simulink model "VVI"  (R2020a)
settings: Solver=FixedStepAuto  StartTime=0.0  StopTime=10.0  FixedStep=1e-3  RelTol=1e-3  EnableMultiTasking=on
undefined symbols (not defined in the file): D0, D1, D10, D11, D12, D13, D2, D3, D4, D5, D6, D7, D8, D9, PTA0, PTA1, PTA2, PTB23, PTB9, PTC16, PTC17, PTC2, PTC3, PTC4, PTD0, PTD1, PTD2, PTD3
libraries: frdmk64flib x15
settings Model: ExtModeTrigDuration=5  Creator=abdullah  LastModifiedBy=abdullah
settings OptimizationCC: EnhancedBackFolding=on  PassReuseOutputArgsAs=Individual arguments  ZeroExternalMemoryAtStartup=off  ZeroInternalMemoryAtStartup=off  MaxStackSize=64  OptimizeBlockOrder=speed  DifferentSizesBufferReuse=on  OptimizationCustomize=off  EfficientTunableParamExpr=on
settings DebuggingCC: ParameterTunabilityLossMsg=error
settings HardwareCC: ProdBitPerPointer=32  ProdBitPerSizeT=32  ProdBitPerPtrDiffT=32  ProdLargestAtomicInteger=Long  ProdLargestAtomicFloat=Double  ProdWordSize=32  ProdHWDeviceType=ARM Compatible->ARM Cortex
settings SFSimCC: MATLABDynamicMemAlloc=off
settings RTWCC: SystemTargetFile=ert.tlc  HardwareBoard=NXP FRDM-K64F  TemplateMakefile=ert_default_tmf  Toolchain=GNU Tools for ARM Embedded Processors
settings CodeAppCC: ForceParamTrailComments=on  IgnoreCustomStorageClasses=off  OperatorAnnotations=on  SimulinkDataObjDesc=on  SFDataObjDesc=on  InsertBlockDesc=on

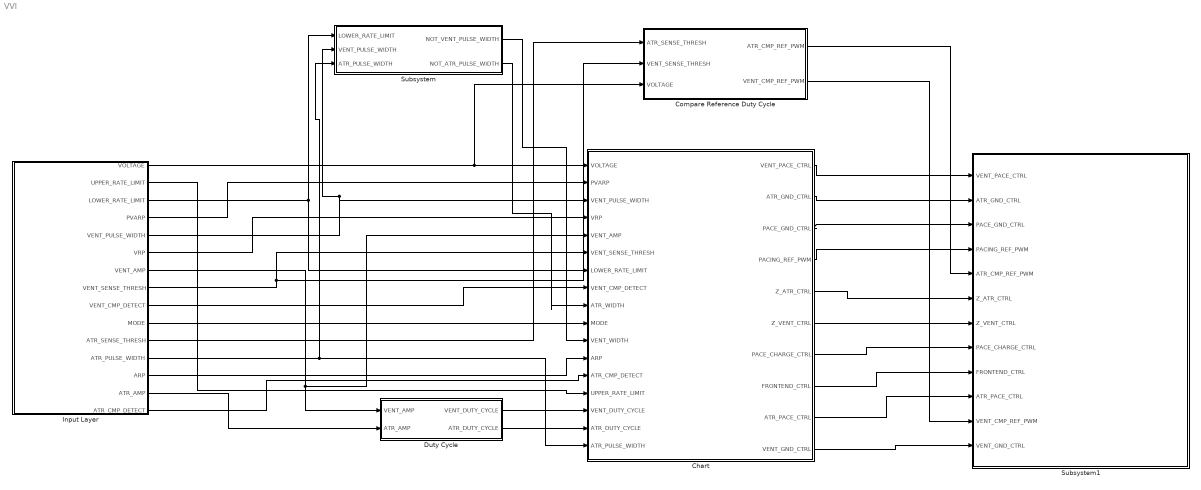
== system VVI ==
  Chart : Stateflow chart  TreatAsAtomicUnit=on
  Compare Reference Duty Cycle : Subsystem
  Duty Cycle : Subsystem
  Input Layer : Subsystem
  Subsystem : Subsystem
  Subsystem1 : Subsystem
  wires:
  Input Layer/1(VOLTAGE) -> Chart/1(VOLTAGE), Compare Reference Duty Cycle/3(VOLTAGE)
  Input Layer/2(UPPER_RATE_LIMIT) -> Chart/14(UPPER_RATE_LIMIT)
  Input Layer/3(LOWER_RATE_LIMIT) -> Subsystem/1(LOWER_RATE_LIMIT), Chart/7(LOWER_RATE_LIMIT)
  Input Layer/4(PVARP) -> Chart/2(PVARP)
  Input Layer/5(VENT_PULSE_WIDTH) -> Subsystem/2(VENT_PULSE_WIDTH), Chart/3(VENT_PULSE_WIDTH)
  Input Layer/6(VRP) -> Chart/4(VRP)
  Input Layer/7(VENT_AMP) -> Duty Cycle/1(VENT_AMP), Chart/5(VENT_AMP)
  Input Layer/8(VENT_SENSE_THRESH) -> Chart/6(VENT_SENSE_THRESH), Compare Reference Duty Cycle/2(VENT_SENSE_THRESH)
  Input Layer/9(VENT_CMP_DETECT) -> Chart/8(VENT_CMP_DETECT)
  Subsystem/1(NOT_VENT_PULSE_WIDTH) -> Chart/11(VENT_WIDTH)
  Chart/1(VENT_PACE_CTRL) -> Subsystem1/1(VENT_PACE_CTRL)
  Chart/2(ATR_GND_CTRL) -> Subsystem1/2(ATR_GND_CTRL)
  Chart/3(PACE_GND_CTRL) -> Subsystem1/3(PACE_GND_CTRL)
  Chart/4(PACING_REF_PWM) -> Subsystem1/4(PACING_REF_PWM)
  Chart/5(Z_ATR_CTRL) -> Subsystem1/6(Z_ATR_CTRL)
  Chart/6(Z_VENT_CTRL) -> Subsystem1/7(Z_VENT_CTRL)
  Chart/7(PACE_CHARGE_CTRL) -> Subsystem1/8(PACE_CHARGE_CTRL)
  Chart/8(FRONTEND_CTRL) -> Subsystem1/9(FRONTEND_CTRL)
  Chart/9(ATR_PACE_CTRL) -> Subsystem1/10(ATR_PACE_CTRL)
  Chart/10(VENT_GND_CTRL) -> Subsystem1/12(VENT_GND_CTRL)
  Duty Cycle/1(VENT_DUTY_CYCLE) -> Chart/15(VENT_DUTY_CYCLE)
  Compare Reference Duty Cycle/1(ATR_CMP_REF_PWM) -> Subsystem1/5(ATR_CMP_REF_PWM)
  Compare Reference Duty Cycle/2(VENT_CMP_REF_PWM) -> Subsystem1/11(VENT_CMP_REF_PWM)
  Input Layer/11(ATR_SENSE_THRESH) -> Compare Reference Duty Cycle/1(ATR_SENSE_THRESH)
  Input Layer/10(MODE) -> Chart/10(MODE)
  Input Layer/12(ATR_PULSE_WIDTH) -> Subsystem/3(ATR_PULSE_WIDTH), Chart/17(ATR_PULSE_WIDTH)
  Subsystem/2(NOT_ATR_PULSE_WIDTH) -> Chart/9(ATR_WIDTH)
  Input Layer/13(ARP) -> Chart/12(ARP)
  Input Layer/14(ATR_AMP) -> Duty Cycle/2(ATR_AMP)
  Duty Cycle/2(ATR_DUTY_CYCLE) -> Chart/16(ATR_DUTY_CYCLE)
  Input Layer/15(ATR_CMP_DETECT) -> Chart/13(ATR_CMP_DETECT)

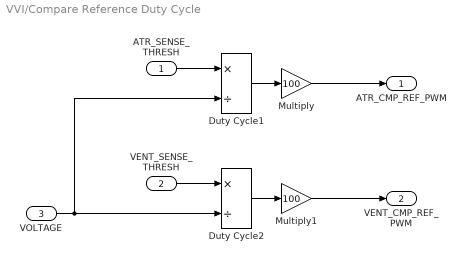
== system VVI/Compare Reference Duty Cycle ==
  ATR_SENSE_THRESH : Inport
  VENT_SENSE_THRESH : Inport  Port=2
  VOLTAGE : Inport  Port=3
  Duty Cycle1 : Product  Inputs=*/
  Duty Cycle2 : Product  Inputs=*/
  Multiply : Gain  Gain=100
  Multiply1 : Gain  Gain=100
  ATR_CMP_REF_PWM : Outport  VectorParamsAs1DForOutWhenUnconnected=off
  VENT_CMP_REF_PWM : Outport  Port=2  VectorParamsAs1DForOutWhenUnconnected=off
  wires:
  Multiply1/1 -> VENT_CMP_REF_PWM/1
  VENT_SENSE_THRESH/1 -> Duty Cycle2/1
  Duty Cycle2/1 -> Multiply1/1
  ATR_SENSE_THRESH/1 -> Duty Cycle1/1
  Duty Cycle1/1 -> Multiply/1
  Multiply/1 -> ATR_CMP_REF_PWM/1
  VOLTAGE/1 -> Duty Cycle1/2, Duty Cycle2/2

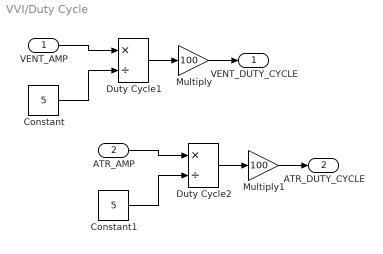
== system VVI/Duty Cycle ==
  VENT_AMP : Inport
  ATR_AMP : Inport  Port=2
  Constant : Constant  Value=5  OutDataTypeStr=single
  Constant1 : Constant  Value=5  OutDataTypeStr=single
  Duty Cycle1 : Product  Inputs=*/
  Duty Cycle2 : Product  Inputs=*/
  Multiply : Gain  Gain=100
  Multiply1 : Gain  Gain=100
  VENT_DUTY_CYCLE : Outport  VectorParamsAs1DForOutWhenUnconnected=off
  ATR_DUTY_CYCLE : Outport  Port=2  VectorParamsAs1DForOutWhenUnconnected=off
  wires:
  Constant/1 -> Duty Cycle1/2
  VENT_AMP/1 -> Duty Cycle1/1
  Duty Cycle1/1 -> Multiply/1
  Multiply/1 -> VENT_DUTY_CYCLE/1
  ATR_AMP/1 -> Duty Cycle2/1
  Multiply1/1 -> ATR_DUTY_CYCLE/1
  Constant1/1 -> Duty Cycle2/2
  Duty Cycle2/1 -> Multiply1/1

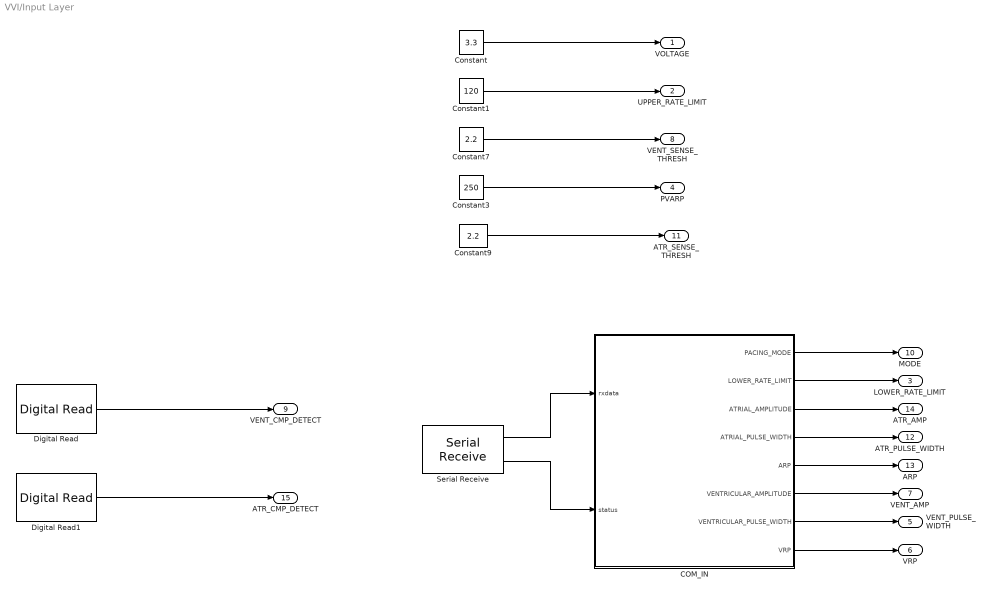
== system VVI/Input Layer ==
  COM_IN : Stateflow chart  TreatAsAtomicUnit=on
  Constant : Constant  Value=3.3  OutDataTypeStr=single
  Constant1 : Constant  Value=120  OutDataTypeStr=uint8
  Constant3 : Constant  Value=250  OutDataTypeStr=uint16
  Constant7 : Constant  Value=2.2  OutDataTypeStr=single
  Constant9 : Constant  Value=2.2  OutDataTypeStr=single
  Digital Read : frdmk64flib/Digital Read  Whichpin=PTC17 (D1)  SampleTime=-1
  Digital Read1 : frdmk64flib/Digital Read  Whichpin=PTC16 (D0)  SampleTime=-1
  Serial Receive : frdmk64flib/Serial Receive  SCIModule=0  Baudrate=uint32(9600)  Parity=None  StopBits=1  HardwareFlowControl=None  ByteOrder=LittleEndian  DataType=uint8  DataLength=24  BlockingMode=off  OutputStatus=on  SampleTime=-1
  VOLTAGE : Outport
  UPPER_RATE_LIMIT : Outport  Port=2
  LOWER_RATE_LIMIT : Outport  Port=3
  PVARP : Outport  Port=4
  VENT_PULSE_WIDTH : Outport  Port=5
  VRP : Outport  Port=6
  VENT_AMP : Outport  Port=7
  VENT_SENSE_THRESH : Outport  Port=8
  VENT_CMP_DETECT : Outport  Port=9
  MODE : Outport  Port=10
  ATR_SENSE_THRESH : Outport  Port=11
  ATR_PULSE_WIDTH : Outport  Port=12
  ARP : Outport  Port=13
  ATR_AMP : Outport  Port=14
  ATR_CMP_DETECT : Outport  Port=15
  wires:
  Serial Receive/1 -> COM_IN/1(rxdata)
  Constant1/1 -> UPPER_RATE_LIMIT/1
  Constant3/1 -> PVARP/1
  Constant/1 -> VOLTAGE/1
  Constant9/1 -> ATR_SENSE_THRESH/1
  Digital Read1/1 -> ATR_CMP_DETECT/1
  Constant7/1 -> VENT_SENSE_THRESH/1
  COM_IN/5(ARP) -> ARP/1
  Digital Read/1 -> VENT_CMP_DETECT/1
  COM_IN/3(ATRIAL_AMPLITUDE) -> ATR_AMP/1
  COM_IN/6(VENTRICULAR_AMPLITUDE) -> VENT_AMP/1
  COM_IN/7(VENTRICULAR_PULSE_WIDTH) -> VENT_PULSE_WIDTH/1
  COM_IN/8(VRP) -> VRP/1
  COM_IN/2(LOWER_RATE_LIMIT) -> LOWER_RATE_LIMIT/1
  COM_IN/4(ATRIAL_PULSE_WIDTH) -> ATR_PULSE_WIDTH/1
  COM_IN/1(PACING_MODE) -> MODE/1
  Serial Receive/2 -> COM_IN/2(status)

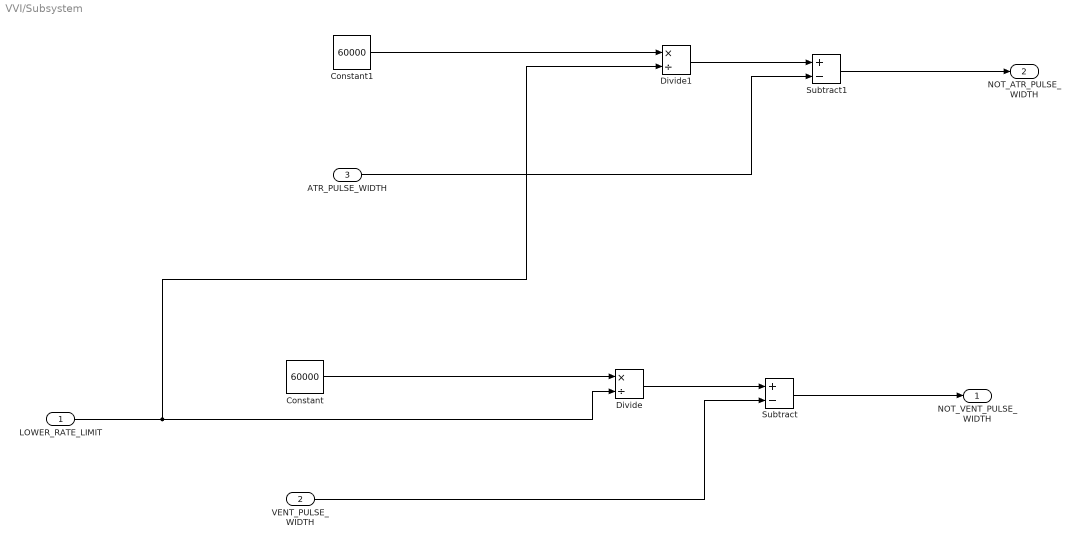
== system VVI/Subsystem ==
  LOWER_RATE_LIMIT : Inport
  VENT_PULSE_WIDTH : Inport  Port=2
  ATR_PULSE_WIDTH : Inport  Port=3
  Constant : Constant  Value=60000
  Constant1 : Constant  Value=60000
  Divide : Product  Inputs=*/
  Divide1 : Product  Inputs=*/
  Subtract : Sum  Inputs=+-  OutDataTypeStr=uint16
  Subtract1 : Sum  Inputs=+-  OutDataTypeStr=uint16
  NOT_VENT_PULSE_WIDTH : Outport
  NOT_ATR_PULSE_WIDTH : Outport  Port=2
  wires:
  LOWER_RATE_LIMIT/1 -> Divide1/2, Divide/2
  Constant/1 -> Divide/1
  Divide/1 -> Subtract/1
  VENT_PULSE_WIDTH/1 -> Subtract/2
  Subtract/1 -> NOT_VENT_PULSE_WIDTH/1
  ATR_PULSE_WIDTH/1 -> Subtract1/2
  Constant1/1 -> Divide1/1
  Divide1/1 -> Subtract1/1
  Subtract1/1 -> NOT_ATR_PULSE_WIDTH/1

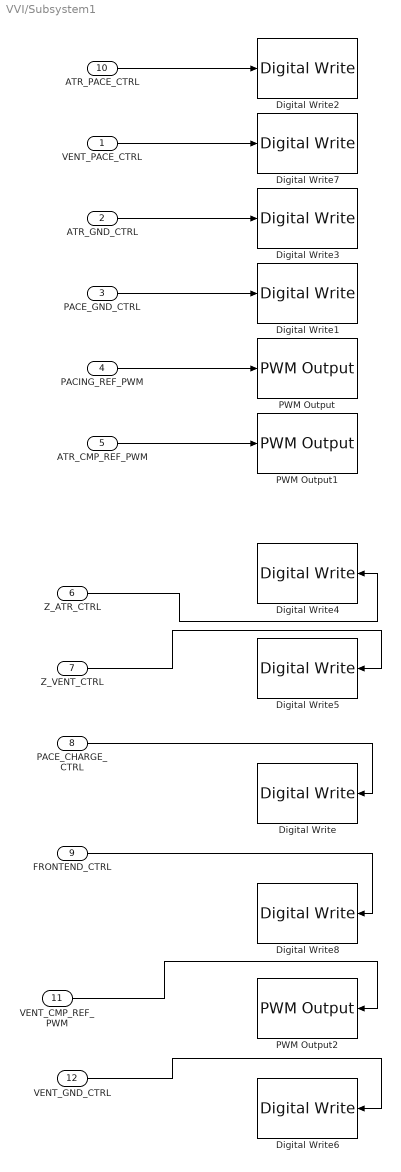
== system VVI/Subsystem1 ==
  VENT_PACE_CTRL : Inport
  ATR_GND_CTRL : Inport  Port=2
  PACE_GND_CTRL : Inport  Port=3
  PACING_REF_PWM : Inport  Port=4
  ATR_CMP_REF_PWM : Inport  Port=5
  Z_ATR_CTRL : Inport  Port=6
  Z_VENT_CTRL : Inport  Port=7
  PACE_CHARGE_CTRL : Inport  Port=8
  FRONTEND_CTRL : Inport  Port=9
  ATR_PACE_CTRL : Inport  Port=10
  VENT_CMP_REF_PWM : Inport  Port=11
  VENT_GND_CTRL : Inport  Port=12
  Digital Write : frdmk64flib/Digital Write  Whichpin=PTB9 (D2)
  Digital Write1 : frdmk64flib/Digital Write  Whichpin=PTD0 (D10)
  Digital Write2 : frdmk64flib/Digital Write  Whichpin=PTA0 (D8)
  Digital Write3 : frdmk64flib/Digital Write  Whichpin=PTD2 (D11)
  Digital Write4 : frdmk64flib/Digital Write  Whichpin=PTB23 (D4)
  Digital Write5 : frdmk64flib/Digital Write  Whichpin=PTC3 (D7)
  Digital Write6 : frdmk64flib/Digital Write  Whichpin=PTD3 (D12)
  Digital Write7 : frdmk64flib/Digital Write  Whichpin=PTC4 (D9)
  Digital Write8 : frdmk64flib/Digital Write  Whichpin=PTD1 (D13)
  PWM Output : frdmk64flib/PWM Output  Whichpin=PTA2 (D5)  InitialFrequency=2000  InitialDutyCycle=30
  PWM Output1 : frdmk64flib/PWM Output  Whichpin=PTC2 (D6)  InitialFrequency=2000  InitialDutyCycle=30
  PWM Output2 : frdmk64flib/PWM Output  Whichpin=PTA1 (D3)  InitialFrequency=2000  InitialDutyCycle=30
  wires:
  PACING_REF_PWM/1 -> PWM Output/1
  ATR_GND_CTRL/1 -> Digital Write3/1
  VENT_PACE_CTRL/1 -> Digital Write7/1
  PACE_GND_CTRL/1 -> Digital Write1/1
  ATR_CMP_REF_PWM/1 -> PWM Output1/1
  Z_ATR_CTRL/1 -> Digital Write4/1
  Z_VENT_CTRL/1 -> Digital Write5/1
  PACE_CHARGE_CTRL/1 -> Digital Write/1
  FRONTEND_CTRL/1 -> Digital Write8/1
  ATR_PACE_CTRL/1 -> Digital Write2/1
  VENT_CMP_REF_PWM/1 -> PWM Output2/1
  VENT_GND_CTRL/1 -> Digital Write6/1

== stateflow chart VVI/Input Layer/COM_IN ==
  settings: executeAtInitialization=1
  state SET_PARAM
    entry:
    PACING_MODE = rxdata(3);
    LOWER_RATE_LIMIT = rxdata(4);
    ATRIAL_AMPLITUDE = typecast(rxdata(5:8), 'single');
    ATRIAL_PULSE_WIDTH = typecast(rxdata(9:12), 'single');
    ARP = typecast(rxdata(13:14), 'uint16');
    VENTRICULAR_AMPLITUDE = typecast(rxdata(15:18), 'single');
    VENTRICULAR_PULSE_WIDTH = typecast(rxdata(19:22), 'single');
    VRP = typecast(rxdata(23:24), 'uint16');
  state INITIAL
    entry:
    PACING_MODE = 1;
    LOWER_RATE_LIMIT = 60;
    ATRIAL_AMPLITUDE = 5;
    ATRIAL_PULSE_WIDTH = 10;
    ARP = 200;
    VENTRICULAR_AMPLITUDE = 5;
    VENTRICULAR_PULSE_WIDTH = 10;
    VRP = 200;
  state STANDBY
    %Waiting for COM
  (default) -> INITIAL
  SET_PARAM -> STANDBY
  (junction 27) -> SET_PARAM [order 2]
  (junction 29) -> SET_PARAM : [rxdata(2) == hex2dec('55')]
  INITIAL -> STANDBY
  STANDBY -> (junction 27) : [status == 0]
  (junction 27) -> (junction 29) [order 1] : [rxdata(1) == hex2dec('16')]
  data: PACING_MODE output uint8; LOWER_RATE_LIMIT output uint8; ATRIAL_AMPLITUDE output single; ATRIAL_PULSE_WIDTH output single; ARP output uint16; VENTRICULAR_AMPLITUDE output single; VENTRICULAR_PULSE_WIDTH output single; VRP output uint16; rxdata input uint8; status input uint8

== stateflow chart VVI/Chart ==
  state INTERMIDIATE
    during:
    PACE_GND_CTRL = true
    VENT_PACE_CTRL = false
    Z_ATR_CTRL = false
    Z_VENT_CTRL = false
    ATR_PACE_CTRL = false
    ATR_GND_CTRL = true
    VENT_GND_CTRL = false
    ATR_PACE_CTRL = false
    VENT_PACE_CTRL = false
    PACING_REF_PWM = ATR_DUTY_CYCLE
    PACE_CHARGE_CTRL = true
  state DISCHARGING3
    during:
    PACE_CHARGE_CTRL = false
    PACE_GND_CTRL = true
    ATR_PACE_CTRL = true
    ATR_GND_CTRL = false
    Z_ATR_CTRL = false
    Z_VENT_CTRL = false
    VENT_GND_CTRL = false
    VENT_PACE_CTRL = false
  state CHARGING3
    during:
    ATR_PACE_CTRL = false
    VENT_PACE_CTRL = false
    PACING_REF_PWM = ATR_DUTY_CYCLE
    PACE_CHARGE_CTRL = true
    PACE_GND_CTRL = true
    VENT_PACE_CTRL = false
    Z_ATR_CTRL = false
    Z_VENT_CTRL = false
    ATR_PACE_CTRL = false
    ATR_GND_CTRL = true
    VENT_GND_CTRL = false
  state CHARGING2
    during:
    ATR_PACE_CTRL = false
    VENT_PACE_CTRL = false
    PACING_REF_PWM = ATR_DUTY_CYCLE
    PACE_CHARGE_CTRL = true
    PACE_GND_CTRL = true
    VENT_PACE_CTRL = false
    Z_ATR_CTRL = false
    Z_VENT_CTRL = false
    ATR_PACE_CTRL = false
    ATR_GND_CTRL = true
    VENT_GND_CTRL = false
  state DISCHARGING2
    during:
    PACE_CHARGE_CTRL = false
    PACE_GND_CTRL = true
    ATR_PACE_CTRL = true
    ATR_GND_CTRL = false
    Z_ATR_CTRL = false
    Z_VENT_CTRL = false
    VENT_GND_CTRL = false
    VENT_PACE_CTRL = false
  state DISCHARGING1
    during:
    PACE_CHARGE_CTRL = false
    PACE_GND_CTRL = true
    ATR_PACE_CTRL = false
    ATR_GND_CTRL = false
    Z_ATR_CTRL = false
    Z_VENT_CTRL = false
    VENT_GND_CTRL = false
    VENT_PACE_CTRL = true
  state CHARGING1
    during:
    ATR_PACE_CTRL = false
    VENT_PACE_CTRL = false
    PACING_REF_PWM = VENT_DUTY_CYCLE
    PACE_CHARGE_CTRL = true
    PACE_GND_CTRL = true
    VENT_PACE_CTRL = false
    Z_ATR_CTRL = false
    Z_VENT_CTRL = false
    ATR_PACE_CTRL = false
    ATR_GND_CTRL = false
    VENT_GND_CTRL = true
  state Start
  state INTERMEDIATE
    during:
    PACE_GND_CTRL = true
    VENT_PACE_CTRL = false
    Z_ATR_CTRL = false
    Z_VENT_CTRL = false
    ATR_PACE_CTRL = false
    ATR_GND_CTRL = false
    VENT_GND_CTRL = true
    ATR_PACE_CTRL = false
    VENT_PACE_CTRL = false
    PACING_REF_PWM = VENT_DUTY_CYCLE
    PACE_CHARGE_CTRL = true
  state CHARGING
    during:
    ATR_PACE_CTRL = false
    VENT_PACE_CTRL = false
    PACING_REF_PWM = VENT_DUTY_CYCLE
    PACE_CHARGE_CTRL = true
    PACE_GND_CTRL = true
    VENT_PACE_CTRL = false
    Z_ATR_CTRL = false
    Z_VENT_CTRL = false
    ATR_PACE_CTRL = false
    ATR_GND_CTRL = false
    VENT_GND_CTRL = true
  state DISCHARGING
    during:
    PACE_CHARGE_CTRL = false
    PACE_GND_CTRL = true
    ATR_PACE_CTRL = false
    ATR_GND_CTRL = false
    Z_ATR_CTRL = false
    Z_VENT_CTRL = false
    VENT_GND_CTRL = false
    VENT_PACE_CTRL = true
  (junction 108) -> INTERMIDIATE : after(VENT_PULSE_WIDTH,msec)
  CHARGING3 -> (junction 108) [order 1] : [ATR_CMP_DETECT == true]
  DISCHARGING3 -> INTERMIDIATE : after(ATR_PULSE_WIDTH, msec)
  INTERMIDIATE -> CHARGING3 : after(ARP, msec)
  CHARGING3 -> Start [order 3] : [MODE~=3]
  Start -> CHARGING3 [order 4] : [MODE==3]
  CHARGING3 -> DISCHARGING3 [order 2] : after(ATR_WIDTH - ARP, msec)
  CHARGING2 -> DISCHARGING2 [order 2] : after(ATR_WIDTH, msec)
  Start -> CHARGING2 [order 3] : [MODE==1]
  DISCHARGING2 -> CHARGING2 : after(ATR_PULSE_WIDTH,msec)
  CHARGING2 -> Start [order 1] : [MODE~=1]
  DISCHARGING1 -> CHARGING1 : after(VENT_PULSE_WIDTH,msec)
  Start -> CHARGING1 [order 1] : [MODE == 2]
  CHARGING1 -> Start [order 2] : [MODE ~= 2]
  CHARGING1 -> DISCHARGING1 [order 1] : after(VENT_WIDTH,msec)
  (default) -> Start
  CHARGING -> Start [order 3] : [MODE~=4]
  Start -> CHARGING [order 2] : [MODE==4]
  (junction 106) -> INTERMEDIATE : after(VENT_PULSE_WIDTH,msec)
  CHARGING -> (junction 106) [order 1] : [VENT_CMP_DETECT == true]
  DISCHARGING -> INTERMEDIATE : after(VENT_PULSE_WIDTH, msec)
  INTERMEDIATE -> CHARGING : after(VRP, msec)
  CHARGING -> DISCHARGING [order 2] : after(VENT_WIDTH - VRP, msec)
  data: VOLTAGE input single; PVARP input uint16; VENT_PULSE_WIDTH input single; VRP input uint16; VENT_AMP input single; VENT_SENSE_THRESH input single; LOWER_RATE_LIMIT input uint8; VENT_CMP_DETECT input boolean; ATR_WIDTH input uint16; MODE input uint8; VENT_WIDTH input uint16; ARP input uint16; ATR_CMP_DETECT input boolean; UPPER_RATE_LIMIT input uint8; VENT_PACE_CTRL output boolean; ATR_GND_CTRL output boolean; PACE_GND_CTRL output boolean; PACING_REF_PWM output single; Z_ATR_CTRL output boolean; Z_VENT_CTRL output boolean; PACE_CHARGE_CTRL output boolean; FRONTEND_CTRL output boolean =true; ATR_PACE_CTRL output boolean; VENT_GND_CTRL output boolean; VENT_DUTY_CYCLE input single; ATR_DUTY_CYCLE input single; ATR_PULSE_WIDTH input single
